simulink model "wind_field_modelling"  (R2020b)
settings: Solver=VariableStepAuto  StartTime=0.0  StopTime=100.0  RelTol=1e-3
libraries: sharedtransform x1
settings Model: Creator=Dogukan  LastModifiedBy=Dogukan

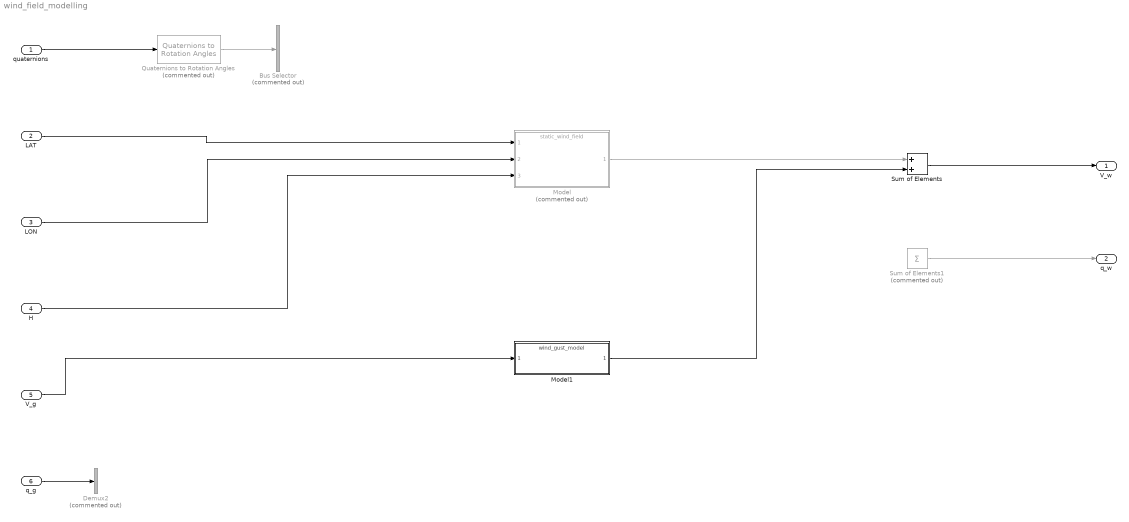
== system wind_field_modelling ==
  quaternions : Inport
  LAT : Inport  Port=2
  LON : Inport  Port=3
  H : Inport  Port=4
  V_g : Inport  Port=5
  q_g : Inport  Port=6
  Bus Selector : BusSelector  Commented=on  OutputSignals=signal1,signal2
  Demux2 : Demux  Commented=on  Outputs=3
  Model : ModelReference  Commented=on  ModelNameDialog=static_wind_field.slx  SimulationMode=Normal  ModelReferenceVersion=1.7
  Model1 : ModelReference  ModelNameDialog=wind_gust_model.slx  SimulationMode=Normal  ModelReferenceVersion=1.1
  Quaternions to Rotation Angles : sharedtransform/Quaternions to Rotation Angles  Commented=on  rotationOrder=ZYX  aMode=aMode
      settings: SourceProductBaseCode=AE,PW,MT,UV,VE,VP
  Sum of Elements : Sum
  Sum of Elements1 : Sum  Commented=on  Inputs=+
  V_w : Outport
  q_w : Outport  Port=2
  wires:
  quaternions/1 -> Quaternions to Rotation Angles/1
  Quaternions to Rotation Angles/1 -> Bus Selector/1
  V_g/1 -> Model1/1
  q_g/1 -> Demux2/1
  LAT/1 -> Model/1
  LON/1 -> Model/2
  H/1 -> Model/3
  Sum of Elements/1 -> V_w/1
  Sum of Elements1/1 -> q_w/1
  Model1/1 -> Sum of Elements/2
  Model/1 -> Sum of Elements/1
